simulink model "planmodel"  (R2025b)
settings: Solver=ode4  StartTime=0.0  StopTime=200  FixedStep=0.001  RelTol=1e-3
values from neighbouring files (symbols this model uses):
  a0 = 340.294    [plan.m]
  b_ref = 2.0    (= 2)    [plan.m]
  c_gear = [0.8e4, 1.4e4, 1.4e4]    [plan.m]
  c_lat = [1.4e4, 2.2e4, 2.2e4]    [plan.m]
  c_ref = 0.9    [plan.m]
  c_roll = [0.020, 0.018, 0.018]    [plan.m]
  CD0 = 0.045    [plan.m]
  CL0 = 0.083    [plan.m]
  CLa = 2.50    (= 2.5)    [plan.m]
  Clb = -0.08    [plan.m]
  Clda = 0.20    (= 0.2)    [plan.m]
  CLde = 0.25    [plan.m]
  Clp = -0.70    (= -0.7)    [plan.m]
  CLq = 3.00    (= 3)    [plan.m]
  Clr = 0    [plan.m]
  Cm0 = 0.112    [plan.m]
  Cma = -0.8    [plan.m]
  Cmde = 0.90    (= 0.9)    [plan.m]
  Cmq = -18.0    (= -18)    [plan.m]
  Cnb = -0.25    [plan.m]
  Cndr = 0.15    [plan.m]
  Cnp = 0    [plan.m]
  Cnr = -0.45    [plan.m]
  CSb = -0.8    [plan.m]
  CSdr = 0.18    [plan.m]
  CSr = 0.15    [plan.m]
  D0 = 800    [plan.m]
  da_max = 25    [plan.m]
  da_min = -da_max    (= -25)    [plan.m]
  de_max = 25    [plan.m]
  de_min = -de_max    (= -25)    [plan.m]
  DH = pi / 180    (= 0.0174532925199)    [plan.m]
  dr_max = 25    [plan.m]
  dr_min = -dr_max    (= -25)    [plan.m]
  g = 9.80665    [plan.m]
  gamma0 = 0.0    (= 0)    [plan.m]
  ground_y = 0.0    (= 0)    [plan.m]
  HD = 180 / pi    (= 57.2957795131)    [plan.m]
  Ixx = 120.0    (= 120)    [plan.m]
  Iyy = 480.0    (= 480)    [plan.m]
  Izz = 520.0    (= 520)    [plan.m]
  K = 0.080    (= 0.08)    [plan.m]
  K_alpha = (wd^2-a24)/(2*zeta*wd)    (= 9.375)    [controller.m]
  k_gear = [1.0e5, 3.0e5, 3.0e5]    [plan.m]
  k_theta0 = 0.0    (= 0)    [plan.m]
  Kb_to_wy = (wd2^2-b24)/(2*zeta*wd2)    [controller.m]
  Kn_pitch = (2.2*wd^2*g)/(Tr*(wd^2-a24)*V_test*a34)    [controller.m]
  Kn_to_beta = (2.2*wd2^2*g)/(Tr*(wd2^2-b24)*V_test*b34)    [controller.m]
  Kw_pitch = -(2*zeta*wd) / a25    [controller.m]
  Kw_to_dr = -2*zeta*wd2/b27    [controller.m]
  m = 600.0    (= 600)    [plan.m]
  mu_brake = [0.0, 0.55, 0.55]    [plan.m]
  omigax0 = 0    [plan.m]
  omigay0 = 0    [plan.m]
  omigaz0 = 0    [plan.m]
  psi0 = 0.0    (= 0)    [plan.m]
  r_left_b = r_gear_b(:,2)    [plan.m]
  r_nose_b = r_gear_b(:,1)    [plan.m]
  r_right_b = r_gear_b(:,3)    [plan.m]
  rho0 = 1.225    [plan.m]
  S_ref = 1.2    [plan.m]
  v_eps = 0.20    (= 0.2)    [plan.m]
  V_min = 1    [plan.m]
  V_test = 200    [controller.m]
  Vx0_b = 0.0    (= 0)    [plan.m]
  Vy0_b = 0.0    (= 0)    [plan.m]
  Vz0_b = 0.0    (= 0)    [plan.m]
  wheel_radius = 0.18    [plan.m]
  WOW_on = 0.000    (= 0)    [plan.m]
  Xg0 = 0.0    (= 0)    [plan.m]
  Yg0 = ground_y + wheel_radius - r_gear_b(2,1) - static_deflection    [plan.m]
  Zg0 = 20.0    (= 20)    [plan.m]
libraries: matrix_library x18, slpidlib x1
(part 3 of 3)

== system planmodel/6DOF-MODEL/动力学/起落架模型/纵向力/Subsystem1/Subsystem ==
  sig_nose : Inport
  sig_left : Inport  Port=2
  sig_right : Inport  Port=3
  u_brake : Inport  Port=4
  Constant2 : Constant  Value=mu_brake
  Demux1 : Demux  Outputs=3
  Gain3 : Gain  Gain=-1
  Product3 : Product  Inputs=4
  Product4 : Product  Inputs=4
  Product5 : Product  Inputs=4
  F_brake_nose : Outport
  F_brake_left : Outport  Port=2
  F_brake_right : Outport  Port=3
  wires:
  [N_nose] -> Product3/1
  Demux1/2 -> Product4/4
  [N_left] -> Product4/1
  Gain3/1 -> Product3/3, Product4/3, Product5/3
  [N_right] -> Product5/1
  Demux1/3 -> Product5/4
  u_brake/1 -> Gain3/1
  Constant2/1 -> Demux1/1
  Demux1/1 -> Product3/4
  sig_right/1 -> Product5/2
  Product3/1 -> F_brake_nose/1
  Product5/1 -> F_brake_right/1
  Product4/1 -> F_brake_left/1
  sig_nose/1 -> Product3/2
  sig_left/1 -> Product4/2

== system planmodel/6DOF-MODEL/动力学/起落架模型/纵向力/Subsystem1/Subsystem1 ==
  sig_nose : Inport
  sig_left : Inport  Port=2
  sig_right : Inport  Port=3
  Constant1 : Constant  Value=c_roll
  Demux : Demux  Outputs=3
  Gain : Gain  Gain=-1
  Gain1 : Gain  Gain=-1
  Gain2 : Gain  Gain=-1
  Product : Product  Inputs=3
  Product1 : Product  Inputs=3
  Product2 : Product  Inputs=3
  F_roll_nose : Outport
  F_roll_left : Outport  Port=2
  F_roll_right : Outport  Port=3
  wires:
  sig_left/1 -> Product1/3
  Demux/2 -> Product1/2
  Gain1/1 -> F_roll_left/1
  Constant1/1 -> Demux/1
  [N_nose] -> Product/1
  [N_left] -> Product1/1
  Product1/1 -> Gain1/1
  Demux/1 -> Product/2
  [N_right] -> Product2/1
  Demux/3 -> Product2/2
  Gain/1 -> F_roll_nose/1
  Product/1 -> Gain/1
  Product2/1 -> Gain2/1
  sig_right/1 -> Product2/3
  Gain2/1 -> F_roll_right/1
  sig_nose/1 -> Product/3

== system planmodel/6DOF-MODEL/动力学/起落架模型/纵向力/Subsystem1/Subsystem2 ==
  In1 : Inport
  Constant5 : Constant  Value=0
  Switch : Switch  Criteria=u2 > Threshold  SaturateOnIntegerOverflow=off  InputSameDT=off
  F_long_nose : Outport
  wires:
  In1/1 -> Switch/1
  Constant5/1 -> Switch/3
  Switch/1 -> F_long_nose/1
  [contact_nose] -> Switch/2

== system planmodel/6DOF-MODEL/动力学/起落架模型/纵向力/Subsystem1/Subsystem3 ==
  In1 : Inport
  Constant5 : Constant  Value=0
  Switch : Switch  Criteria=u2 > Threshold  SaturateOnIntegerOverflow=off  InputSameDT=off
  F_long_left : Outport
  wires:
  In1/1 -> Switch/1
  Constant5/1 -> Switch/3
  Switch/1 -> F_long_left/1
  [contact_left] -> Switch/2

== system planmodel/6DOF-MODEL/动力学/起落架模型/纵向力/Subsystem1/Subsystem4 ==
  In1 : Inport
  Constant5 : Constant  Value=0
  Switch : Switch  Criteria=u2 > Threshold  SaturateOnIntegerOverflow=off  InputSameDT=off
  F_long_right : Outport
  wires:
  [contact_right] -> Switch/2
  Switch/1 -> F_long_right/1
  Constant5/1 -> Switch/3
  In1/1 -> Switch/1

== matlab function planmodel/6DOF-MODEL/动力学/起落架模型/侧向力/Subsystem/MATLAB Function1 ==
  data: gamma input; R_gb output; theta input; psi input
function R_gb = ground2body(gamma, theta, psi)
    T1=[cos(psi), 0 ,-sin(psi);...
          0     , 1 ,    0   ;...
        sin(psi), 0 ,cos(psi);];%绕y偏航
    T2=[cos(theta),sin(theta),0;...
        -sin(theta),cos(theta),0;...
          0        , 0 ,       1;];%绕z俯仰角
    T3=[1,0,0;...
        0,cos(gamma),sin(gamma);...
        0,-sin(gamma),cos(gamma);];%绕x滚转角

   R_gb=T3*T2*T1;

== matlab function planmodel/6DOF-MODEL/动力学/起落架模型/侧向力/Subsystem/主轮侧向方向向量 ==
  data: Cbg input; eg_long output; eb_long input
function eg_long= project_long(Cbg,eb_long)


e_y=[0;1;0];
P_g=eye(3)-e_y*e_y';

eg_long=P_g*Cbg*eb_long;
eg_long=eg_long/norm(eg_long);

== matlab function planmodel/6DOF-MODEL/动力学/起落架模型/侧向力/Subsystem/前轮侧向向量 ==
  data: Cbg input; eg_long output; eb_long input
function eg_long= project_long(Cbg,eb_long)


e_y=[0;1;0];
P_g=eye(3)-e_y*e_y';

eg_long=P_g*Cbg*eb_long;
eg_long=eg_long/norm(eg_long);

== matlab function planmodel/6DOF-MODEL/动力学/起落架模型/MATLAB Function1 ==
  data: gamma input; R_gb output; theta input; psi input
function R_gb = ground2body(gamma, theta, psi)
    T1=[cos(psi), 0 ,-sin(psi);...
          0     , 1 ,    0   ;...
        sin(psi), 0 ,cos(psi);];%绕y偏航
    T2=[cos(theta),sin(theta),0;...
        -sin(theta),cos(theta),0;...
          0        , 0 ,       1;];%绕z俯仰角
    T3=[1,0,0;...
        0,cos(gamma),sin(gamma);...
        0,-sin(gamma),cos(gamma);];%绕x滚转角

   R_gb=T3*T2*T1;

== matlab function planmodel/6DOF-MODEL/动力学/起落架模型/MATLAB Function2 ==
  data: gamma input; R_gb output; theta input; psi input
function R_gb = ground2body(gamma, theta, psi)
    T1=[cos(psi), 0 ,-sin(psi);...
          0     , 1 ,    0   ;...
        sin(psi), 0 ,cos(psi);];%绕y偏航
    T2=[cos(theta),sin(theta),0;...
        -sin(theta),cos(theta),0;...
          0        , 0 ,       1;];%绕z俯仰角
    T3=[1,0,0;...
        0,cos(gamma),sin(gamma);...
        0,-sin(gamma),cos(gamma);];%绕x滚转角

   R_gb=T3*T2*T1;

== matlab function planmodel/6DOF-MODEL/动力学/起落架模型/三轮在地系下的力/摩擦圆限幅/前轮摩擦圆限幅 ==
  data: N input; F_long_out output; F_long input; F_lat input; F_lat_out output
function [F_long_out,F_lat_out]=Dround_saturation_nose(N,F_long,F_lat)
mu=0.65;
F_ALL=sqrt((F_long)^2+(F_lat)^2);
if(F_ALL<=mu*N)
    F_long_out=F_long;
    F_lat_out=F_lat;
else
    s=mu*N/F_ALL;
    F_long_out=s*F_long;
    F_lat_out=s*F_lat;
end

== matlab function planmodel/6DOF-MODEL/动力学/起落架模型/三轮在地系下的力/摩擦圆限幅/主轮摩擦圆限幅左 ==
  data: N input; F_long_out output; F_long input; F_lat input; F_lat_out output
function [F_long_out,F_lat_out]=Dround_saturation_main(N,F_long,F_lat)
mu=0.7;
F_ALL=sqrt((F_long)^2+(F_lat)^2);
if(F_ALL<=mu*N)
    F_long_out=F_long;
    F_lat_out=F_lat;
else
    s=mu*N/F_ALL;
    F_long_out=s*F_long;
    F_lat_out=s*F_lat;
end

== matlab function planmodel/6DOF-MODEL/动力学/起落架模型/三轮在地系下的力/摩擦圆限幅/主轮摩擦圆限幅右 ==
  data: N input; F_long_out output; F_long input; F_lat input; F_lat_out output
function [F_long_out,F_lat_out]=Dround_saturation_main(N,F_long,F_lat)
mu=0.7;
F_ALL=sqrt((F_long)^2+(F_lat)^2);
if(F_ALL<=mu*N)
    F_long_out=F_long;
    F_lat_out=F_lat;
else
    s=mu*N/F_ALL;
    F_long_out=s*F_long;
    F_lat_out=s*F_lat;
end

== matlab function planmodel/control/俯仰通道控制器/MATLAB Function ==
  settings: updateMethod=DISCRETE
  data: Vx input; theta_cmd output; no_contact input; t input; theta_actual input
function theta_cmd = fcn(Vx, no_contact, t, theta_actual)
% 起飞抬前轮俯仰角指令生成
% Vx:           机体系前向速度 (m/s)
% no_contact:   无轮接地信号, 1=空中, 0=地面
% t:            仿真时间 (s), 接 Digital Clock
% theta_actual: 飞机当前的实际俯仰角 (rad), 用于离地无缝切换

persistent t_rotation
persistent theta_takeoff_hold

if isempty(t_rotation)
    t_rotation = inf;
end
if isempty(theta_takeoff_hold)
    theta_takeoff_hold = 0;
end

%% --- 参数配置
VR = 65;                      % m/s, 抬轮速度 
theta_target = 4 * pi/180;   % rad,
rotation_rate = 0.5 * pi/180;   % rad/s

%% --- 状态机控制逻辑 ---
if no_contact > 0.5
    % 【空中阶段】
    % 刚离地瞬间，记录下离地时的实际姿态，防止指令断崖式下掉
    if theta_takeoff_hold == 0
        theta_takeoff_hold = theta_actual; 
    end

    theta_cmd = theta_takeoff_hold; 
    
    % 重置滑跑计时器
    t_rotation = inf;

elseif Vx >= VR
    % 【抬轮阶段】
    if isinf(t_rotation)
        t_rotation = t;       % 记录开始抬轮的绝对时间
    end
    
    % 按照设定的速率（3°/s）线性增加俯仰角指令
    theta_cmd = rotation_rate * (t - t_rotation);
    
    % 达到目标角度（10°）后进行限幅切顶
    if theta_cmd > theta_target
        theta_cmd = theta_target;
    end
    
    % 尚未离地，清空离地保持值
    theta_takeoff_hold = 0;

else
    % 【地面加速滑跑阶段】
    % 保持前轮三点接地姿态（通常为 0° 或略微带一点下俯角压前轮，视安装角而定）
    theta_cmd = -10*pi/180; 
    t_rotation = inf;
    theta_takeoff_hold = 0;
end% 在你的状态机逻辑中添加：

end

== matlab function planmodel/6DOF-MODEL/动力学/体系旋转角速度/MATLAB Function ==
  data: alpha input; R_wind_b output; beta input
 function R_wind_b = wind2body(alpha, beta)
T1 = [cos(beta), 0, -sin(beta);
       0, 1, 0;
       sin(beta), 0, cos(beta)];
T2 = [cos(alpha), sin(alpha), 0;
       -sin(alpha), cos(alpha), 0;
       0, 0, 1];
R_wind_b = T2*T1;

== matlab function planmodel/6DOF-MODEL/动力学/Subsystem3/MATLAB Function1 ==
  data: gamma input; R_gb output; theta input; psi input
function R_gb = ground2body(gamma, theta, psi)
    T1=[cos(psi), 0 ,-sin(psi);...
          0     , 1 ,    0   ;...
        sin(psi), 0 ,cos(psi);];%绕y偏航
    T2=[cos(theta),sin(theta),0;...
        -sin(theta),cos(theta),0;...
          0        , 0 ,       1;];%绕z俯仰角
    T3=[1,0,0;...
        0,cos(gamma),sin(gamma);...
        0,-sin(gamma),cos(gamma);];%绕x滚转角

   R_gb=T3*T2*T1;

== matlab function planmodel/6DOF-MODEL/动力学/起落架模型/起落架三轮质心在地系下位置/MATLAB Function1 ==
  data: gamma input; R_gb output; theta input; psi input
function R_gb = ground2body(gamma, theta, psi)
    T1=[cos(psi), 0 ,-sin(psi);...
          0     , 1 ,    0   ;...
        sin(psi), 0 ,cos(psi);];%绕y偏航
    T2=[cos(theta),sin(theta),0;...
        -sin(theta),cos(theta),0;...
          0        , 0 ,       1;];%绕z俯仰角
    T3=[1,0,0;...
        0,cos(gamma),sin(gamma);...
        0,-sin(gamma),cos(gamma);];%绕x滚转角

   R_gb=T3*T2*T1;

== matlab function planmodel/6DOF-MODEL/动力学/height/MATLAB Function2 ==
  data: gamma input; R_gb output; theta input; psi input
function R_gb = ground2body(gamma, theta, psi)
    T1=[cos(psi), 0 ,-sin(psi);...
          0     , 1 ,    0   ;...
        sin(psi), 0 ,cos(psi);];%绕y偏航
    T2=[cos(theta),sin(theta),0;...
        -sin(theta),cos(theta),0;...
          0        , 0 ,       1;];%绕z俯仰角
    T3=[1,0,0;...
        0,cos(gamma),sin(gamma);...
        0,-sin(gamma),cos(gamma);];%绕x滚转角

   R_gb=T3*T2*T1;

== matlab function planmodel/6DOF-MODEL/动力学/v在体系下的分量/MATLAB Function ==
  data: alpha input; R_wind_b output; beta input
 function R_wind_b = wind2body(alpha, beta)
T1 = [cos(beta), 0, -sin(beta);
       0, 1, 0;
       sin(beta), 0, cos(beta)];
T2 = [cos(alpha), sin(alpha), 0;
       -sin(alpha), cos(alpha), 0;
       0, 0, 1];
R_wind_b = T2*T1;

== matlab function planmodel/6DOF-MODEL/动力学/v在体系下的分量/MATLAB Function1 ==
  data: gamma input; R_gb output; theta input; psi input
function R_gb = ground2body(gamma, theta, psi)
    T1=[cos(psi), 0 ,-sin(psi);...
          0     , 1 ,    0   ;...
        sin(psi), 0 ,cos(psi);];%绕y偏航
    T2=[cos(theta),sin(theta),0;...
        -sin(theta),cos(theta),0;...
          0        , 0 ,       1;];%绕z俯仰角
    T3=[1,0,0;...
        0,cos(gamma),sin(gamma);...
        0,-sin(gamma),cos(gamma);];%绕x滚转角

   R_gb=T3*T2*T1;

== matlab function planmodel/6DOF-MODEL/动力学/起落架模型/法向支反力/MATLAB Function1 ==
  data: gamma input; R_gb output; theta input; psi input
function R_gb = ground2body(gamma, theta, psi)
    T1=[cos(psi), 0 ,-sin(psi);...
          0     , 1 ,    0   ;...
        sin(psi), 0 ,cos(psi);];%绕y偏航
    T2=[cos(theta),sin(theta),0;...
        -sin(theta),cos(theta),0;...
          0        , 0 ,       1;];%绕z俯仰角
    T3=[1,0,0;...
        0,cos(gamma),sin(gamma);...
        0,-sin(gamma),cos(gamma);];%绕x滚转角

   R_gb=T3*T2*T1;

== matlab function planmodel/6DOF-MODEL/动力学/起落架模型/纵向力/Subsystem/MATLAB Function1 ==
  data: gamma input; R_gb output; theta input; psi input
function R_gb = ground2body(gamma, theta, psi)
    T1=[cos(psi), 0 ,-sin(psi);...
          0     , 1 ,    0   ;...
        sin(psi), 0 ,cos(psi);];%绕y偏航
    T2=[cos(theta),sin(theta),0;...
        -sin(theta),cos(theta),0;...
          0        , 0 ,       1;];%绕z俯仰角
    T3=[1,0,0;...
        0,cos(gamma),sin(gamma);...
        0,-sin(gamma),cos(gamma);];%绕x滚转角

   R_gb=T3*T2*T1;

== matlab function planmodel/6DOF-MODEL/动力学/起落架模型/纵向力/Subsystem/前轮滚动方向向量 ==
  data: Cbg input; eg_long output; eb_long input
function eg_long= project_long(Cbg,eb_long)

e_y=[0;1;0];
P_g=eye(3)-e_y*e_y';
eg_long=P_g*Cbg*eb_long;
eg_long=eg_long/norm(eg_long);

== matlab function planmodel/6DOF-MODEL/动力学/起落架模型/纵向力/Subsystem/主轮滚动方向向量 ==
  data: Cbg input; eg_long output; eb_long input
function eg_long= project_long(Cbg,eb_long)


e_y=[0;1;0];
P_g=eye(3)-e_y*e_y';

eg_long=P_g*Cbg*eb_long;
eg_long=eg_long/norm(eg_long);
